simulink model "lab4"  (R2025b)
settings: Solver=ode4  StartTime=0.0  StopTime=10.0  FixedStep=2^-7  RelTol=1e-3
libraries: simulink x1
settings Model: Creator=mizula  LastModifiedBy=mizula

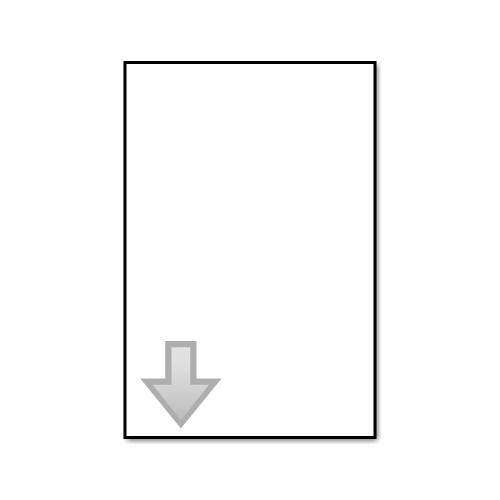
[thumbnail: Simulink's stored preview of the top-level diagram]
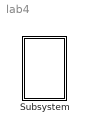
== system lab4 ==
  Subsystem : Subsystem  mask{M=200, R=2, Rs=0.2, G=9.81, x=0, y=5, Vx=20, Vy=7}

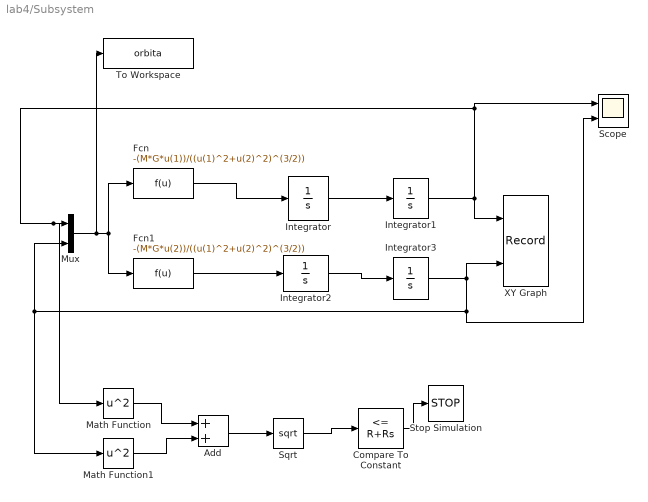
== system lab4/Subsystem ==
  Add : Sum
  Compare To Constant : simulink/Logic and Bit Operations/Compare To Constant  relop=<=  const=R+Rs  OutDataTypeStr=boolean
  Fcn : Fcn  Expr=-(M*G*u(1))/((u(1)^2+u(2)^2)^(3/2))
  Fcn1 : Fcn  Expr=-(M*G*u(2))/((u(1)^2+u(2)^2)^(3/2))
  Integrator : Integrator  InitialCondition=Vx
  Integrator1 : Integrator  InitialCondition=x
  Integrator2 : Integrator  InitialCondition=Vy
  Integrator3 : Integrator  InitialCondition=y
  Math Function : Math  Operator=square
  Math Function1 : Math  Operator=square
  Mux : Mux  Inputs=2
  Scope : Scope  NumInputPorts=2
      settings: ActiveDisplayYMinimum=-24.99924263557449  ActiveDisplayYMaximum=83.072062012981377
  Sqrt : Sqrt
  Stop Simulation : Stop
  To Workspace : ToWorkspace  VariableName=orbita  SaveFormat=Timeseries  SampleTime=-1
  XY Graph : Record  NumPorts=2.0  FileSettingsInternal="{\"entries\":[{\"content\":{\"excelSettings\":{\"content\":{},\"type\":\"Streamout.ExcelSettings\"},\"parquetSettings\":{\"content\":{},\"type\":\"Streamout.ParquetSettings\"}},\"type\":\"Streamout.FileSettingStorage\",\"uuid\":\"\"}],\"packageUris\":[\"http:\\/\\/schema.mathworks.com\\/mf0\\/streamout_blocks\\/R2020a\"],\"version\":\"1.0\"}"  FrameSettings=[0, 0]  Layout=[1 1]  SignalsInternal="{\"entries\":[{\"content\":{\"signals\":[{\"content\":{\"blockPath\":[],\"dimensions\":[1],\"domain\":\"\",\"lineColor\":\"#a2142f\",\"plots\":[ 1 ],\"port\":1,\"sid\":[\"\"],\"signalID\":1,\"signalName\":\"Integrator1\"},\"type\":\"RecordBlkView.Signal\",\"uuid\":\"\"},{\"content\":{\"blockPath\":[],\"dimensions\":[1],\"domain\":\"\",\"lineColor\":\"#139fff\",\"plots\":[ 1 ],\"port\":2,\"sid\":[\"\"],\"signalID\":2,\"signalName\":\"Integrator3\"},\"type\":\"RecordBlkView.Signal\",\"uuid\":\"\"}]},\"type\":\"RecordBlkView.InputSignals\",\"uuid\":\"\"}],\"packageUris\":[\"http:\\/\\/schema.mathworks.com\\/mf0\\/streamout_blocks\\/R2020a\"],\"version\":\"1.0\"}"  VisualizationBindings="{\"xyplotplugin\":{\"info\":[{\"series\":[{\"bindingParametersList\":[{\"parameter\":\"X-Axis\",\"signalID\":1,\"signalName\":\"Integrator1\"},{\"parameter\":\"Y-Axis\",\"signalID\":2,\"signalName\":\"Integrator3\"}],\"seriesID\":0}],\"subplotID\":1}]}}"  CompatibilityTag=XY
  wires:
  Integrator/1 -> Integrator1/1
  Fcn/1 -> Integrator/1
  Mux/1 -> To Workspace/1, Fcn/1, Fcn1/1
  Fcn1/1 -> Integrator2/1
  Math Function/1 -> Add/1
  Compare To Constant/1 -> Stop Simulation/1
  Add/1 -> Sqrt/1
  Integrator3/1 -> XY Graph/2, Scope/2, Math Function1/1, Mux/2
  Integrator2/1 -> Integrator3/1
  Integrator1/1 -> XY Graph/1, Scope/1, Math Function/1, Mux/1
  Sqrt/1 -> Compare To Constant/1
  Math Function1/1 -> Add/2
